simulink model "impedance"  (R2021b)
settings: Solver=VariableStepAuto  StartTime=0.0  StopTime=5  RelTol=1e-3
undefined symbols (not defined in the file): invMd, K, Kd, Kp, Md, xr
libraries: robotcorelib x1, simulink x1
settings Model: Creator=fabio  LastModifiedBy=buse

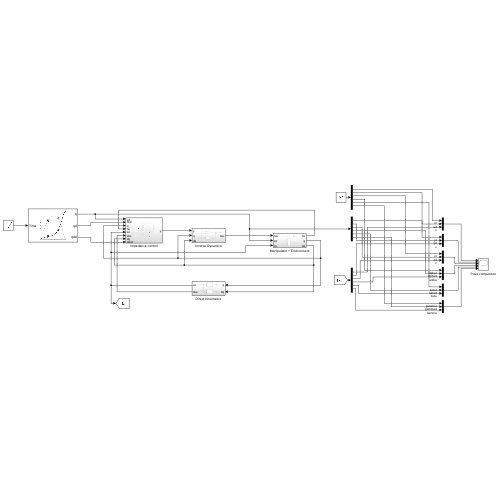
[thumbnail: Simulink's stored preview of the top-level diagram]
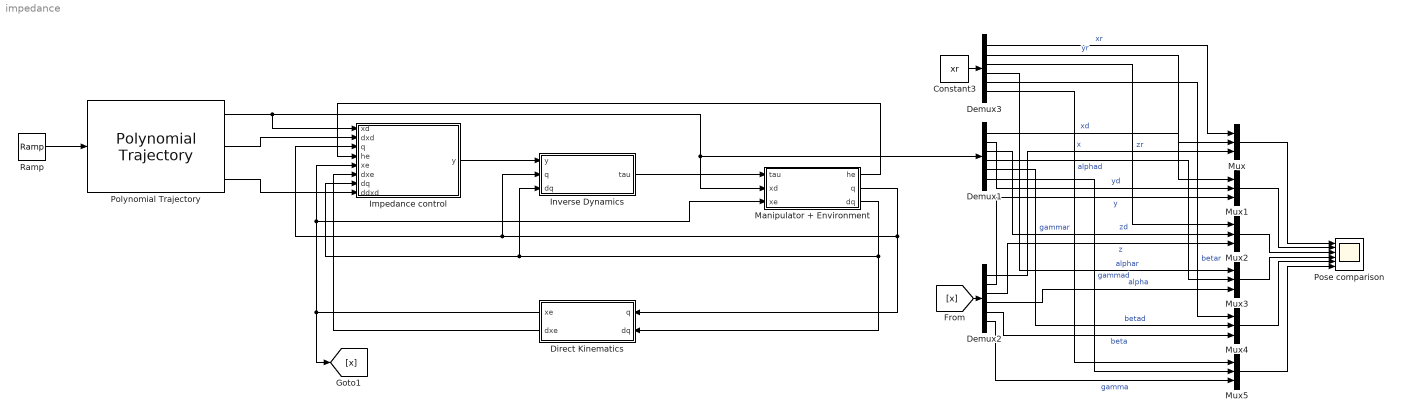
== system impedance ==
  Constant3 : Constant  Value=xr
  Demux1 : Demux  Outputs=6
  Demux2 : Demux  Outputs=6
  Demux3 : Demux  Outputs=6
  Direct Kinematics : Subsystem
  Impedance control : Subsystem
  Inverse Dynamics : Subsystem
  Manipulator + Environment : Subsystem
  Mux{,1..5} (6 alike) : Mux  Inputs=3
  Polynomial Trajectory : robotcorelib/Polynomial Trajectory  WaypointSource=Internal  Waypoints=op_wpts  TimePoints=time  TimeInterval=[ 1, 4 ]  Method=Quintic Polynomial  ParameterSource=Internal  VelocityBoundaryCondition=velBound  AccelerationBoundaryCondition=accBound  SimulateUsing=Interpreted execution
  Pose comparison : Scope  NumInputPorts=6
  Ramp : simulink/Sources/Ramp  slope=1  start=0  InitialOutput=0
  wires:
  Mux1/1 -> Pose comparison/2
  Demux1/4 -> Mux3/2  "alphad"
  Demux1/1 -> Mux/2  "xd"
  Mux4/1 -> Pose comparison/5
  Demux2/1 -> Mux/3  "x"
  Demux1/3 -> Mux2/2  "zd"
  Demux2/4 -> Mux3/3  "alpha"
  Demux1/6 -> Mux5/2  "gammad"
  Demux2/2 -> Mux1/3  "y"
  Mux/1 -> Pose comparison/1
  Demux2/3 -> Mux2/3  "z"
  Polynomial Trajectory/1 -> Impedance control/1(xd), Demux1/1, Manipulator + Environment/2(xd)
  Mux3/1 -> Pose comparison/4
  Demux2/5 -> Mux4/3  "beta"
  Demux1/2 -> Mux1/2  "yd"
  Demux1/5 -> Mux4/2  "betad"
  Mux5/1 -> Pose comparison/6
  Mux2/1 -> Pose comparison/3
  [x] -> Demux2/1
  Demux2/6 -> Mux5/3  "gamma"
  Constant3/1 -> Demux3/1
  Demux3/1 -> Mux/1  "xr"
  Demux3/2 -> Mux1/1  "yr"
  Demux3/3 -> Mux2/1  "zr"
  Demux3/4 -> Mux3/1  "alphar"
  Demux3/5 -> Mux4/1  "betar"
  Demux3/6 -> Mux5/1  "gammar"
  Manipulator + Environment/1(he) -> Impedance control/4(he)
  Manipulator + Environment/2(q) -> Inverse Dynamics/2(q), Impedance control/3(q), Direct Kinematics/1(q)
  Direct Kinematics/1(xe) -> [x], Impedance control/5(xe), Manipulator + Environment/3(xe)
  Impedance control/1(y) -> Inverse Dynamics/1(y)
  Inverse Dynamics/1(tau) -> Manipulator + Environment/1(tau)
  Direct Kinematics/2(dxe) -> Impedance control/6(dxe)
  Manipulator + Environment/3(dq) -> Direct Kinematics/2(dq), Impedance control/7(dq), Inverse Dynamics/3(dq)
  Ramp/1 -> Polynomial Trajectory/1
  Polynomial Trajectory/2 -> Impedance control/2(dxd)
  Polynomial Trajectory/3 -> Impedance control/8(ddxd)

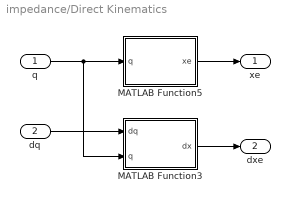
== system impedance/Direct Kinematics ==
  q : Inport
  dq : Inport  Port=2
  MATLAB Function3 : MATLAB Function  TreatAsAtomicUnit=on
  MATLAB Function5 : MATLAB Function  TreatAsAtomicUnit=on
  xe : Outport
  dxe : Outport  Port=2
  wires:
  MATLAB Function3/1(dx) -> dxe/1
  q/1 -> MATLAB Function3/2(q), MATLAB Function5/1(q)
  MATLAB Function5/1(xe) -> xe/1
  dq/1 -> MATLAB Function3/1(dq)

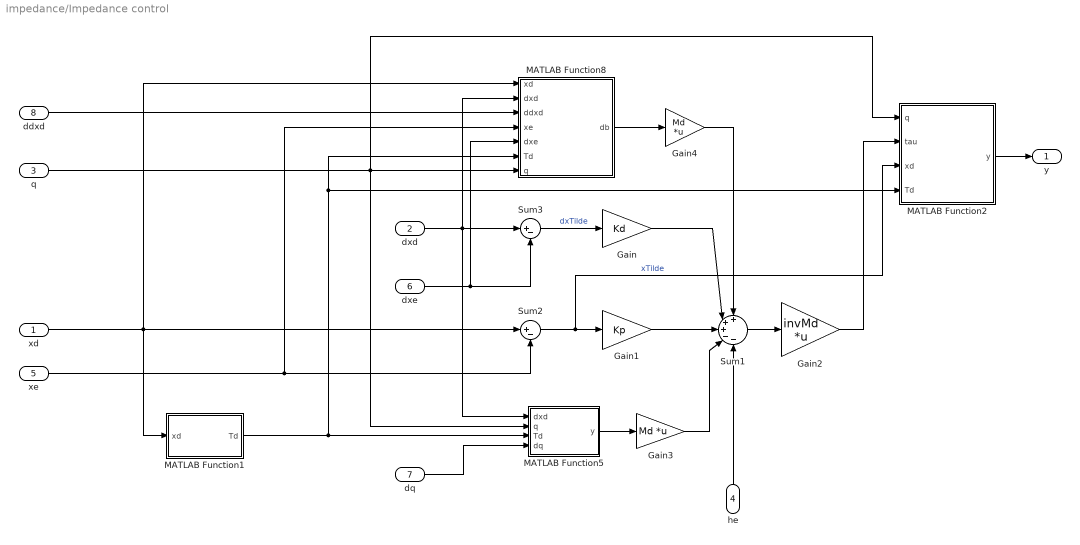
== system impedance/Impedance control ==
  xd : Inport
  dxd : Inport  Port=2
  q : Inport  Port=3
  he : Inport  Port=4
  xe : Inport  Port=5
  dxe : Inport  Port=6
  dq : Inport  Port=7
  ddxd : Inport  Port=8
  Gain : Gain  Gain=Kd
  Gain1 : Gain  Gain=Kp
  Gain2 : Gain  Gain=invMd  Multiplication=Matrix(K*u)
  Gain3 : Gain  Gain=Md  Multiplication=Matrix(K*u)
  Gain4 : Gain  Gain=Md  Multiplication=Matrix(K*u)
  MATLAB Function1 : MATLAB Function  TreatAsAtomicUnit=on
  MATLAB Function2 : MATLAB Function  TreatAsAtomicUnit=on
  MATLAB Function5 : MATLAB Function  TreatAsAtomicUnit=on
  MATLAB Function8 : MATLAB Function  TreatAsAtomicUnit=on
  Sum1 : Sum  Inputs=+++--
  Sum2 : Sum  Inputs=|+-
  Sum3 : Sum  Inputs=|+-
  y : Outport
  wires:
  MATLAB Function1/1(Td) -> MATLAB Function5/3(Td), MATLAB Function2/4(Td), MATLAB Function8/6(Td)
  MATLAB Function8/1(db) -> Gain4/1
  MATLAB Function5/1(y) -> Gain3/1
  Gain2/1 -> MATLAB Function2/2(tau)
  dxd/1 -> MATLAB Function8/2(dxd), MATLAB Function5/1(dxd), Sum3/1
  xd/1 -> MATLAB Function1/1(xd), MATLAB Function8/1(xd), Sum2/1
  Gain3/1 -> Sum1/4
  MATLAB Function2/1(y) -> y/1
  Gain/1 -> Sum1/2
  Sum3/1 -> Gain/1  "dxTilde"
  Sum1/1 -> Gain2/1
  Gain1/1 -> Sum1/3
  Gain4/1 -> Sum1/1
  q/1 -> MATLAB Function2/1(q), MATLAB Function5/2(q), MATLAB Function8/7(q)
  xe/1 -> MATLAB Function8/4(xe), Sum2/2
  dxe/1 -> Sum3/2, MATLAB Function8/5(dxe)
  dq/1 -> MATLAB Function5/4(dq)
  ddxd/1 -> MATLAB Function8/3(ddxd)
  Sum2/1 -> MATLAB Function2/3(xd), Gain1/1  "xTilde"
  he/1 -> Sum1/5

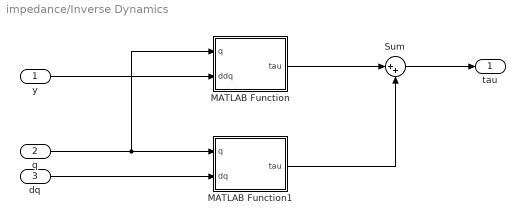
== system impedance/Inverse Dynamics ==
  y : Inport
  q : Inport  Port=2
  dq : Inport  Port=3
  MATLAB Function : MATLAB Function  TreatAsAtomicUnit=on
  MATLAB Function1 : MATLAB Function  TreatAsAtomicUnit=on
  Sum : Sum  Inputs=|++
  tau : Outport
  wires:
  MATLAB Function1/1(tau) -> Sum/2
  MATLAB Function/1(tau) -> Sum/1
  Sum/1 -> tau/1
  dq/1 -> MATLAB Function1/2(dq)
  q/1 -> MATLAB Function/1(q), MATLAB Function1/1(q)
  y/1 -> MATLAB Function/2(ddq)

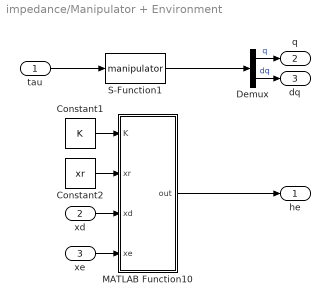
== system impedance/Manipulator + Environment ==
  tau : Inport
  xd : Inport  Port=2
  xe : Inport  Port=3
  Constant1 : Constant  Value=K
  Constant2 : Constant  Value=xr
  Demux : Demux  Outputs=2
  MATLAB Function10 : MATLAB Function  TreatAsAtomicUnit=on
  S-Function1 : S-Function  FunctionName=manipulator  Parameters=robot  SFunctionDeploymentMode=off  EnableBusSupport=off
  he : Outport
  q : Outport  Port=2
  dq : Outport  Port=3
  wires:
  tau/1 -> S-Function1/1
  Constant1/1 -> MATLAB Function10/1(K)
  Constant2/1 -> MATLAB Function10/2(xr)
  xd/1 -> MATLAB Function10/3(xd)
  xe/1 -> MATLAB Function10/4(xe)
  S-Function1/1 -> Demux/1
  Demux/1 -> q/1  "q"
  Demux/2 -> dq/1  "dq"
  MATLAB Function10/1(out) -> he/1

== matlab function impedance/Inverse Dynamics/MATLAB Function1 ==
  data: q input size=3; tau output; dq input size=3
function tau = N(q, dq)
    q1 = q(1); q2 = q(2); q3 = q(3);
    dq1 = dq(1); dq2 = dq(2); dq3 = dq(3);
    tau = [dq3*(0.03923*cos(q3)*dq3^2 - 0.5*dq1*(0.0474*sin(2.0*q3) + 0.05885*sin(q3) + 0.1962*q2*sin(q3))*dq3) - 1.0*dq1*(0.5*dq3^2*(0.0474*sin(2.0*q3) + 0.05885*sin(q3) + 0.1962*q2*sin(q3)) - 0.5*dq2^2*(3.098*q2 + 0.1962*cos(q3) + 0.7099)) + 0.5*dq1*dq2^2*(3.098*q2 + 0.1962*cos(q3) + 0.7099);
            0.5*dq1^2*dq2*(3.098*q2 + 0.1962*cos(q3) + 0.7099);
            dq1*(0.03923*cos(q3)*dq3^2 - 0.5*dq1*(0.0474*sin(2.0*q3) + 0.05885*sin(q3) + 0.1962*q2*sin(q3))*dq3) - 0.9621*cos(q3)];
end

== matlab function impedance/Inverse Dynamics/MATLAB Function ==
  data: q input size=3; tau output; ddq input size=3
function tau = B(q, ddq)
    q1 = q(1); q2 = q(2); q3 = q(3);
    B = getB(q,0);
    tau = B*ddq;

== matlab function impedance/Impedance control/MATLAB Function1 ==
  data: xd input; Td output
function Td = getTd(xd)
    % Euler angles -> rotation matrix  
    s1 = sin(xd(4)); s2 = sin(xd(5)); s3 = sin(xd(6));
    c1 = cos(xd(4)); c2 = cos(xd(5)); c3 = cos(xd(6));
    Rd = [ c1*c3-c2*s1*s3, -c1*s3-c2*c3*s1, s1*s2;
           c3*s1+c1*c2*s3, c1*c2*c3-s1*s3, -c1*s2;
           s2*s3, c3*s2, c2
        ];
    % Extract the translation vector
    t = xd(1:3);
    Td = [Rd t
        zeros(1,3) 1];

== matlab function impedance/Direct Kinematics/MATLAB Function3 ==
  data: dq input; dx output; q input
function dx = JA(dq, q)
    q1 = q(1); q2 = q(2); q3 = q(3);
    JA =[(3*cos(q1))/10 - (2*sin(q1))/5 + (6*cos(q1)*cos(q3))/25 + q2*cos(q1),  sin(q1), -(6*sin(q1)*sin(q3))/25;
        (2*cos(q1))/5 + (3*sin(q1))/10 + (6*cos(q3)*sin(q1))/25 + q2*sin(q1), -cos(q1),  (6*cos(q1)*sin(q3))/25;
        0,        0,          (6*cos(q3))/25;
        1,        0,                       0;
        0,        0,                      -1;
        0,        0,                       0]; 
    dx = JA*dq;

== matlab function impedance/Direct Kinematics/MATLAB Function5 ==
  data: q input size=3; xe output size=6
function xe = k(q)
    q1 = q(1); q2 = q(2); q3 = q(3);
    % Direct kinematics
    xe = [(2*cos(q1))/5 + (3*sin(q1))/10 + (6*cos(q3)*sin(q1))/25 + q2*sin(q1);
         (2*sin(q1))/5 - (3*cos(q1))/10 - (6*cos(q1)*cos(q3))/25 - q2*cos(q1);
         (6*sin(q3))/25 + 3/20;
         q1;
         pi/2 - q3;
         pi/2];

== matlab function impedance/Impedance control/MATLAB Function2 ==
  data: q input; y output; tau input; xd input; Td input
function y = invJad(q, tau, xd, Td)
    q1 = q(1); q2 = q(2); q3 = q(3);
    % Base to ee transformation matrix
    Te = [-sin(q1)*sin(q3), -cos(q1),  cos(q3)*sin(q1), (2*cos(q1))/5 + (3*sin(q1))/10 + (6*cos(q3)*sin(q1))/25 + q2*sin(q1);
     cos(q1)*sin(q3), -sin(q1), -cos(q1)*cos(q3), (2*sin(q1))/5 - (3*cos(q1))/10 - (6*cos(q1)*cos(q3))/25 - q2*cos(q1);
             cos(q3),        0,          sin(q3),                                                (6*sin(q3))/25 + 3/20;
                   0,        0,                0,                                                                    1];
    % Td frame to ee transformation matrix
    Tde = Td/Te;
    % pinv(Ta(Phi))
    Ta = [
        [1, 0, 0, 0,       0, 0]
        [0, 1, 0, 0,       0, 0]
        [0, 0, 1, 0,       0, 0]
        [0, 0, 0, 0,       0, 1]  
        [0, 0, 0, cos(q1), sin(q1), 0]
        [0, 0, 0, 0, 0, 0]
    ];
    J = [
[(3*cos(q1))/10 - (2*sin(q1))/5 + (6*cos(q1)*cos(q3))/25 + q2*cos(q1),  sin(q1), -(6*sin(q1)*sin(q3))/25]
[(2*cos(q1))/5 + (3*sin(q1))/10 + (6*cos(q3)*sin(q1))/25 + q2*sin(q1), -cos(q1),  (6*cos(q1)*sin(q3))/25]
[                                                                   0,        0,          (6*cos(q3))/25]
[                                                                   0,        0,                -cos(q1)]
[                                                                   0,        0,                -sin(q1)]
[                                                                   1,        0,                       0]
 ];
    % Euler angles -> rotation matrix  
    s1 = sin(xd(4)); s2 = sin(xd(5)); s3 = sin(xd(6));
    c1 = cos(xd(4)); c2 = cos(xd(5)); c3 = cos(xd(6));
    Rd = [ c1*c3-c2*s1*s3, -c1*s3-c2*c3*s1, s1*s2;
           c3*s1+c1*c2*s3, c1*c2*c3-s1*s3, -c1*s2;
           s2*s3, c3*s2, c2
        ];
    % R matrix slide 14 
    R = [Rd' zeros(3,3)
        zeros(3,3) Rd'];
    jad = (Ta*R*J);
    y = pinv(jad)*tau;

== matlab function impedance/Impedance control/MATLAB Function5 ==
  data: dxd input; q input; Td input; y output; dq input
function y = dJadq(dxd, q, Td,dq)
    q1 = q(1); q2 = q(2); q3 = q(3);
    dq1 = dq(1); dq2 = dq(2); dq3 = dq(3);
    % Base to ee transformation matrix
    Te = [-sin(q1)*sin(q3), -cos(q1),  cos(q3)*sin(q1), (2*cos(q1))/5 + (3*sin(q1))/10 + (6*cos(q3)*sin(q1))/25 + q2*sin(q1);
     cos(q1)*sin(q3), -sin(q1), -cos(q1)*cos(q3), (2*sin(q1))/5 - (3*cos(q1))/10 - (6*cos(q1)*cos(q3))/25 - q2*cos(q1);
             cos(q3),        0,          sin(q3),                                                (6*sin(q3))/25 + 3/20;
                   0,        0,                0,                                                                    1];
    % Td frame to ee transformation matrix
    Tde = Td/Te;
    % pinv(Ta)
    invTa = [
        [1, 0, 0,          0,          0, 0]
        [0, 1, 0,          0,          0, 0]
        [0, 0, 1,          0,          0, 0]
        [0, 0, 0,          0,          0, 1]
        [0, 0, 0, cos(q1), sin(q1), 0]
        [0, 0, 0,          0,          0, 0]
    ];     
    J = [
        [(3*cos(q1))/10 - (2*sin(q1))/5 + (6*cos(q1)*cos(q3))/25 + q2*cos(q1),  sin(q1), -(6*sin(q1)*sin(q3))/25]
        [(2*cos(q1))/5 + (3*sin(q1))/10 + (6*cos(q3)*sin(q1))/25 + q2*sin(q1), -cos(q1),  (6*cos(q1)*sin(q3))/25]
        [                                                                   0,        0,          (6*cos(q3))/25]
        [                                                                   0,        0,                -cos(q1)]
        [                                                                   0,        0,                -sin(q1)]
        [                                                                   1,        0,                       0]
    ];    
    dJ = [
        [dq2*cos(q1) - (2*dq1*cos(q1))/5 - (3*dq1*sin(q1))/10 - dq1*sin(q1)*q2 - (6*dq1*cos(q3)*sin(q1))/25 - (6*dq3*cos(q1)*sin(q3))/25, dq1*cos(q1), - (6*dq1*cos(q1)*sin(q3))/25 - (6*dq3*cos(q3)*sin(q1))/25]
        [(3*dq1*cos(q1))/10 - (2*dq1*sin(q1))/5 + dq2*sin(q1) + (6*dq1*cos(q1)*cos(q3))/25 - (6*dq3*sin(q1)*sin(q3))/25 + dq1*cos(q1)*q2, dq1*sin(q1),   (6*dq3*cos(q1)*cos(q3))/25 - (6*dq1*sin(q1)*sin(q3))/25]
        [                                                                                                                                                         0,              0,                                                -(6*dq3*sin(q3))/25]
        [                                                                                                                                                         0,              0,                                                        dq1*sin(q1)]
        [                                                                                                                                                         0,              0,                                                       -dq1*cos(q1)]
        [                                                                                                                                                         0,              0,                                                                     0]
    ];   
    
    Rdt = Td(1:3, 1:3)';    
    wd = dxd(4:6);   
    swd=[0 -wd(3) wd(2)
        wd(3) 0 -wd(1)
        -wd(2) wd(1) 0 ];    
    RdMat = [Rdt zeros(3);zeros(3) Rdt];    
    dJad = invTa*([Rdt*swd zeros(3);zeros(3) Rdt*swd]*J+RdMat*dJ); % invDTa = 0
    y = dJad*dq;

== matlab function impedance/Impedance control/MATLAB Function8 ==
  data: xd input; dxd input; ddxd input; xe input; dxe input; db output; Td input; q input
function db = diffB(xd,dxd,ddxd,xe,dxe, Td,q)
    % Slide 29
    q1 = q(1); q2 = q(2); q3 = q(3);
    %Rotation Matrix
    Rdt = Td(1:3, 1:3)';
    %Desired pos
    od = xd(1:3);
    %Desired vel
    dod = dxd(1:3);
    wd = dxd(4:6);
    %Desired acc
    ddod = ddxd(1:3);
    dwd = ddxd(4:6);
    %Pos end effector
    oe = xe(1:3);
    %Vel end effector
    doe = dxe(1:3);
    swd=[0 -wd(3) wd(2)
        wd(3) 0 -wd(1)
        -wd(2) wd(1) 0 ];
    sdwd=[0 -dwd(3) dwd(2)
        dwd(3) 0 -dwd(1)
        -dwd(2) dwd(1) 0 ];
    db = [
        Rdt*swd*dod+Rdt*ddod+Rdt*sdwd*(od-oe)+Rdt*swd*(dod-doe); 0; 0; 0 % invDT = 0
    ];

== matlab function impedance/Manipulator + Environment/MATLAB Function10 ==
  data: K input; out output size=6; xr input; xd input; xe input size=6
function out = he(K, xr, xd, xe)
    he = zeros(6,1);
    if xe(2) > xr(2) % Only along y, i.e. only when moving only joint 2
        % In contact
        dxrd = xd-xr;
        dxed = xd-xe;
        dxre = dxrd-dxed;
        he = K*dxre;
    end
    % Equilibrium point
    out = he;
